simulink model "p1_digital_twin_R2023a"  (R2023a)
settings: Solver=FixedStepDiscrete  StartTime=0.0  StopTime=10  FixedStep=Ts  RelTol=1e-3  EnableMultiTasking=on
values from neighbouring files (symbols this model uses):
  ack = 1    [SteeringController.m]
  cpr_handwheel = 500*4    (= 2000)    [p1_params_new.m]
  cpr_steering = 1000*4    (= 4000)    [p1_params_new.m]
  hal_filter_den = [1 1*(2*pi*Ts)-1]    [SteeringController.m]    (also in p1_params_new.m = DEN_cellarray{1})
  hal_filter_num = [1*(2*pi*Ts)]    [SteeringController.m]    (also in p1_params_new.m = NUM_cellarray{1})
  n_drive = 5.6    [p1_params_new.m]
  n_handwheel = 50    [p1_params_new.m]
  n_steering = 160    [p1_params_new.m]
  sr = 7.5    [SteeringController.m]
  steering_limit = 35    [SteeringController.m]
  Ts = 0.001    [p1_params_new.m]
  wc = 10    [SteeringController.m]    (also in p1_params_new.m = p1params.input.VAccelFc*(2*Ts))
undefined symbols (not defined in the file or in its folder): DiscIntNeverNeededParam, p1params, param
libraries: simulink x7
(part 1 of 4)
settings Model: ExtModeTrigDuration=2  Creator=cbeal  LastModifiedBy=12406
settings SolverCC: InitialStep=.001  ZeroCrossAlgorithm=Adaptive  AlgebraicLoopSolver=TrustRegion  PositivePriorityOrder=on
settings DataIOCC: SaveFormat=Array  SignalLoggingSaveFormat=ModelDataLogs  SignalLogging=off  ReturnWorkspaceOutputs=off  Refine=5
settings OptimizationCC: EnhancedBackFolding=on  PassReuseOutputArgsAs=Individual arguments  ExpressionDepthLimit=2147483647  ZeroExternalMemoryAtStartup=off  ZeroInternalMemoryAtStartup=off  MaxStackSize=64  OptimizeBlockOrder=speed  DifferentSizesBufferReuse=on  OptimizationCustomize=off  EfficientTunableParamExpr=on
settings DebuggingCC: UnderspecifiedInitializationDetection=Classic  MergeDetectMultiDrivingBlocksExec=none  InheritedTsInSrcMsg=none  ParameterTunabilityLossMsg=error  FcnCallInpInsideContextMsg=warning  UnconnectedInputMsg=warning  UnconnectedOutputMsg=warning  UnconnectedLineMsg=warning  StateNameClashWarn=warning  SFUnexpectedBacktrackingDiag=warning  SFNoUnconditionalDefaultTransitionDiag=warning  ArithmeticOperatorsInVariantConditions=warning
settings HardwareCC: ProdBitPerPointer=32  ProdBitPerSizeT=32  ProdBitPerPtrDiffT=32  ProdLargestAtomicInteger=Long  ProdLargestAtomicFloat=Double  ProdWordSize=32  ProdLongLongMode=on  ProdHWDeviceType=ARM Compatible->ARM Cortex
settings ModelReferenceCC: EnableRefExpFcnMdlSchedulingChecks=on  PropagateSignalLabelsOutOfModel=off
settings SFSimCC: SimUseLocalCustomCode=off  CustomCodeUndefinedFunction=UseInterfaceOnly
settings RTWCC: Description=Embedded Coder  SystemTargetFile=ert.tlc  HardwareBoard=Raspberry Pi  TLCOptions="-aInlineSetEventsForThisBaseRateFcn=TLC_FALSE -aSuppressMultiTaskScheduler=TLC_FALSE  -aRateBasedStepFcn=0"  TemplateMakefile=ert_default_tmf  RTWUseLocalCustomCode=off  Toolchain=GNU GCC Embedded Linux  BuildConfiguration=Faster Runs
settings CodeAppCC: ForceParamTrailComments=on  IgnoreCustomStorageClasses=off  OperatorAnnotations=on  SimulinkDataObjDesc=on  SFDataObjDesc=on  InsertBlockDesc=on
settings ERTTargetCC: SupportVariableSizeSignals=on  ExtModeTransport=2  ExtModeStaticAlloc=on  ExtModeMexFile=ext_xcp  ExtModeIntrfLevel=Level2 - Open
settings ConfigComp: CovMetricSettings=dw  CovSaveCumulativeToWorkspaceVar=on  CovSaveSingleToWorkspaceVar=on  CovExternalEMLEnable=off

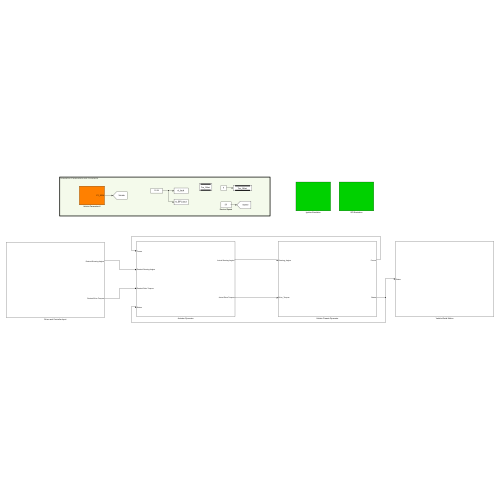
[thumbnail: Simulink's stored preview of the top-level diagram]
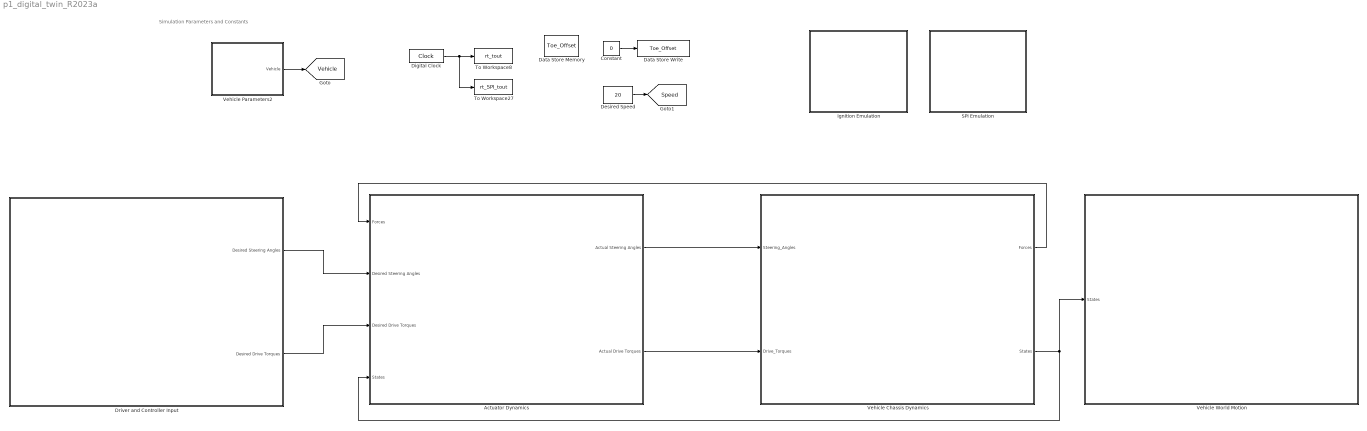
== system p1_digital_twin_R2023a ==
  note: Simulation Parameters and Constants
  Actuator Dynamics : Subsystem
  Constant : Constant  Value=0
  Data Store Memory : DataStoreMemory  DataStoreName=Toe_Offset  WriteAfterWriteMsg=warning  ShowAdditionalParam=off
  Data Store Write : DataStoreWrite  DataStoreName=Toe_Offset  IndexOptions=Index vector (dialog)  Indices=1  OutputSizes=1
  Desired Speed : Constant  Value=20
  Digital Clock : DigitalClock  SampleTime=-1
  Driver and Controller Input : Subsystem
  Ignition Emulation : Subsystem
  SPI Emulation : Subsystem
  To Workspace27 : ToWorkspace  VariableName=rt_SPI_tout  SampleTime=-1
      settings: Save2DSignal=2-D array (concatenate along first dimension)
  To Workspace8 : ToWorkspace  VariableName=rt_tout  SampleTime=-1
      settings: Save2DSignal=2-D array (concatenate along first dimension)
  Vehicle Chassis Dynamics : Subsystem
  Vehicle Parameters2 : Subsystem  mask{vehicleName='P1_2024', m=1467, m_s=1467, Ixx=0, Iyy=0, Izz=2235, Iw=1.2, Re=0.32, a=1.02, b=1.45, d=1.3, h_cg=0.42, h_rcf=0, h_rcr=0, k_phi=0, b_phi=0, Ca=[50000; 50000; 35000; 35000], Cx=[30000; 30000; 30000; 30000], mu_peak=[1.2 1.2 1.2 1.2], mu_slide=[0.9 0.9 0.9 0.9]}
      mask prompts: vehicleName "Name of Vehicle"; m "Mass"; m_s "Sprung Mass"; Ixx "Roll Moment of Inertia"; Iyy "Pitch Moment of Inertia"; Izz "Yaw Moment of Inertia"; Iw "Wheel Moment of Inertia"; Re "Wheel Effective Radius"; a "CG-Front Axle Distance"; b "CG-Rear Axle Distance"; d "Track Width"; h_cg "CG height"; h_rcf "Front Roll Center Height"; h_rcr "Rear Roll Center Height"; k_phi "Chassis Roll Stiffness (x2)"; b_phi "Chassis Roll Damping (x2)"; Ca "Cornering Stiffnesses (x4)"; Cx "Longitudinal Stiffnesses (x4)"; mu_peak "Peak Coeff. Friction (x4)"; mu_slide "Sliding Coeff. Friction (x4)"
      mask Display: port_label('output',1,vehicleName)
  Vehicle World Motion : Subsystem
  tag scope: Speed=global, Vehicle=global
  wires:
  Vehicle Parameters2/1(Vehicle) -> [Vehicle]
  Digital Clock/1 -> To Workspace27/1, To Workspace8/1
  Desired Speed/1 -> [Speed]
  Driver and Controller Input/1(Desired Steering Angles) -> Actuator Dynamics/2(Desired Steering Angles)
  Driver and Controller Input/2(Desired Drive Torques) -> Actuator Dynamics/3(Desired Drive Torques)
  Constant/1 -> Data Store Write/1
  Actuator Dynamics/1(Actual Steering Angles) -> Vehicle Chassis Dynamics/1(Steering_Angles)
  Vehicle Chassis Dynamics/2(States) -> Actuator Dynamics/4(States), Vehicle World Motion/1(States)
  Vehicle Chassis Dynamics/1(Forces) -> Actuator Dynamics/1(Forces)
  Actuator Dynamics/2(Actual Drive Torques) -> Vehicle Chassis Dynamics/2(Drive_Torques)

== system p1_digital_twin_R2023a/Actuator Dynamics ==
  Forces : Inport
  Desired Steering Angles : Inport  Port=2
  Desired Drive Torques : Inport  Port=3
  States : Inport  Port=4
  Bus Selector : BusSelector  OutputSignals=Fy
  Bus Selector1 : BusSelector  OutputSignals=Yaw Rate
  Constant : Constant  Value=0
  Drivetrain Emulation : Subsystem
  Left Steering Model : Subsystem
  Mux : Mux
  Right Steering Model : Subsystem
  Selector : Selector  InputPortWidth=4  IndexOptions=Index vector (dialog)  Indices=[1]  OutputSizes=1
  Selector1 : Selector  InputPortWidth=4  IndexOptions=Index vector (dialog)  Indices=2  OutputSizes=1
  Steering System Emulation : Subsystem
  Actual Steering Angles : Outport
  Actual Drive Torques : Outport  Port=2
  wires:
  Right Steering Model/1(delta_right) -> Mux/2  "Right"
  Left Steering Model/2(steering_left) -> Steering System Emulation/1(Left Wheel)
  Right Steering Model/2(steering_right) -> Steering System Emulation/2(Right Wheel)
  Selector/1 -> Left Steering Model/2(In2)
  Selector1/1 -> Right Steering Model/2(In2)
  Desired Steering Angles/1 -> Selector1/1, Selector/1
  Left Steering Model/1(delta_left) -> Mux/1  "Left"
  Constant/1 -> Mux/4, Mux/3
  Mux/1 -> Actual Steering Angles/1
  Bus Selector/1 -> Right Steering Model/1(Fy), Left Steering Model/1(Fy)  "<Fy>"
  Desired Drive Torques/1 -> Actual Drive Torques/1
  [Speed] -> Drivetrain Emulation/1(Vehicle Speed)
  Forces/1 -> Bus Selector/1
  States/1 -> Bus Selector1/1
  Bus Selector1/1 -> Drivetrain Emulation/2(Vehicle Yaw Rate)  "<Yaw Rate>"

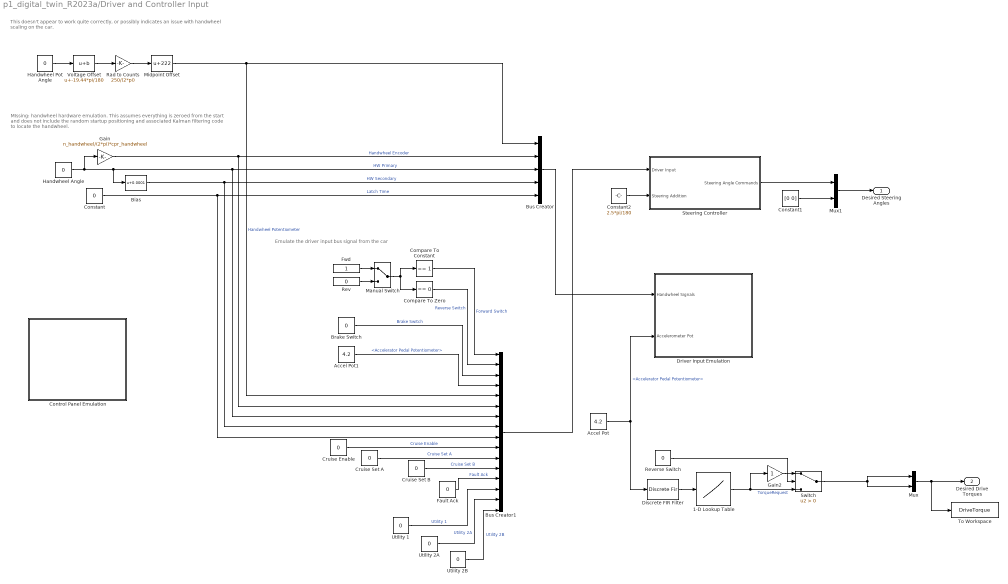
== system p1_digital_twin_R2023a/Driver and Controller Input ==
  note: Emulate the driver input bus signal from the car
  note: This doesn't appear to work quite correctly, or possibly indicates
      | an issue with handwheel scaling on the car.
  note: MIssing: handwheel hardware emulation. This assumes
      | everything is zeroed from the start and does not include the
      | random startup positioning and associated Kalman filtering
      | code to locate the handwheel.
  1-D Lookup Table : Lookup_n-D  NumberOfTableDimensions=1  BreakpointsForDimension1="[0 p1params.input.VminAccel p1params.input.VmidAccel-p1params.input.Vdeadband/2  p1params.input.VmidAccel+p1params.input.Vdeadband/2 p1params.input.VmaxAccel 5]"  Table=[p1params.input.TmaxAccel p1params.input.TmaxAccel 0 0 p1params.input.TminAccel p1params.input.TminAccel]  InternalRulePriority=Speed  RndMeth=Simplest
  Accel Pot : Constant  Value=4.2
  Accel Pot1 : Constant  Value=4.2
  Bias : Bias  Bias=0.0001  SaturateOnIntegerOverflow=off
  Brake Switch : Constant  Value=0
  Bus Creator : BusCreator  Inputs=5
  Bus Creator1 : BusCreator  Inputs=16
  Compare To Constant : simulink/Logic and Bit Operations/Compare To Constant  relop===  const=1  OutDataTypeStr=uint8
  Compare To Zero : simulink/Logic and Bit Operations/Compare To Zero  relop===  OutDataTypeStr=uint8
  Constant : Constant  Value=0
  Constant1 : Constant  Value=[0 0]
  Constant2 : Constant  Value=2.5*pi/180
  Control Panel Emulation : Subsystem
  Cruise Enable : Constant  Value=0
  Cruise Set A : Constant  Value=0
  Cruise Set B : Constant  Value=0
  Discrete FIR Filter : DiscreteFir  Coefficients=[ones(1,20)/20]
  Driver Input Emulation : Subsystem
  Fault Ack : Constant  Value=0
  Fwd : Constant
  Gain : Gain  Gain=n_handwheel/(2*pi)*cpr_handwheel
  Gain2 : Gain
  Handwheel Angle : Constant  Value=0
  Handwheel Pot Angle : Constant  Value=0
  Manual Switch : ManualSwitch
  Midpoint Offset : Bias  Bias=222  SaturateOnIntegerOverflow=off
  Mux : Mux  Inputs=2
  Mux1 : Mux  Inputs=2
  Rad to Counts : Gain  Gain=250/(2*pi)
  Rev : Constant  Value=0
  Reverse Switch : Constant  Value=0
  Steering Controller : Subsystem
      mask init:
      | p1_params_new;
      | SteeringController;
  Switch : Switch  Criteria=u2 > Threshold  SaturateOnIntegerOverflow=off  InputSameDT=off
  To Workspace : ToWorkspace  VariableName=DriveTorque  SampleTime=-1
      settings: Save2DSignal=2-D array (concatenate along first dimension)
  Utility 1 : Constant  Value=0
  Utility 2A : Constant  Value=0
  Utility 2B : Constant  Value=0
  Voltage Offset : Bias  Bias=-19.44*pi/180  SaturateOnIntegerOverflow=off
  Desired Steering Angles : Outport
  Desired Drive Torques : Outport  Port=2
  wires:
  Bus Creator/1 -> Driver Input Emulation/1(Handwheel Signals)
  Constant/1 -> Bus Creator1/9, Bus Creator/5  "Latch Time"
  Midpoint Offset/1 -> Bus Creator1/5, Bus Creator/1  "Handwheel Potentiometer"
  Handwheel Angle/1 -> Bus Creator1/7, Bus Creator/3, Bias/1, Gain/1  "HW Primary"
  Voltage Offset/1 -> Rad to Counts/1
  Handwheel Pot Angle/1 -> Voltage Offset/1
  Bias/1 -> Bus Creator1/8, Bus Creator/4  "HW Secondary"
  Rad to Counts/1 -> Midpoint Offset/1
  Gain/1 -> Bus Creator1/6, Bus Creator/2  "Handwheel Encoder"
  Mux1/1 -> Desired Steering Angles/1
  1-D Lookup Table/1 -> Switch/3, Gain2/1  "TorqueRequest"
  Reverse Switch/1 -> Switch/2
  Accel Pot/1 -> Discrete FIR Filter/1, Driver Input Emulation/2(Accelerometer Pot)  "<Accelerator Pedal Potentiometer>"
  Gain2/1 -> Switch/1
  Discrete FIR Filter/1 -> 1-D Lookup Table/1
  Mux/1 -> To Workspace/1, Desired Drive Torques/1
  Switch/1 -> Mux/2, Mux/1
  Constant1/1 -> Mux1/2
  Constant2/1 -> Steering Controller/2(Steering Addition)
  Steering Controller/1(Steering Angle Commands) -> Mux1/1
  Bus Creator1/1 -> Steering Controller/1(Driver Input)
  Fwd/1 -> Manual Switch/1
  Rev/1 -> Manual Switch/2
  Manual Switch/1 -> Compare To Zero/1, Compare To Constant/1
  Brake Switch/1 -> Bus Creator1/3  "Brake Switch"
  Accel Pot1/1 -> Bus Creator1/4  "<Accelerator Pedal Potentiometer>"
  Utility 2B/1 -> Bus Creator1/16  "Utility 2B"
  Utility 2A/1 -> Bus Creator1/15  "Utility 2A"
  Utility 1/1 -> Bus Creator1/14  "Utility 1"
  Fault Ack/1 -> Bus Creator1/13  "Fault Ack"
  Cruise Set B/1 -> Bus Creator1/12  "Cruise Set B"
  Cruise Set A/1 -> Bus Creator1/11  "Cruise Set A"
  Cruise Enable/1 -> Bus Creator1/10  "Cruise Enable"
  Compare To Zero/1 -> Bus Creator1/2  "Reverse Switch"
  Compare To Constant/1 -> Bus Creator1/1  "Forward Switch"

== system p1_digital_twin_R2023a/Ignition Emulation ==
  note: This is just a single signal that comes from the MCU. It will always
      | be on if we're taking data, so emulate it as a constant 1.
  Constant : Constant  OutDataTypeStr=uint8  SampleTime=-1
  To Workspace22 : ToWorkspace  VariableName=rt_Ignition  SampleTime=-1
      settings: Save2DSignal=2-D array (concatenate along first dimension)
  wires:
  Constant/1 -> To Workspace22/1

== system p1_digital_twin_R2023a/SPI Emulation ==
  note: Since we are not actually receiving anything over SPI in this
      | model, generate random data so that the error checking doesn't
      | flag the rest of the data as repeated (and thus erroneous).
  Constant : Constant  Value=rand(215,1)  OutDataTypeStr=double  SampleTime=-1
  Data Type Conversion : DataTypeConversion  OutDataTypeStr=uint8  SaturateOnIntegerOverflow=off  RndMeth=Floor
  Gain : Gain  Gain=255  OutDataTypeStr=double  SaturateOnIntegerOverflow=on
  Round : Rounding
  To Workspace17 : ToWorkspace  VariableName=rt_spiBytesIn  SampleTime=-1
      settings: Save2DSignal=2-D array (concatenate along first dimension)
  wires:
  Constant/1 -> Gain/1
  Round/1 -> Data Type Conversion/1
  Gain/1 -> Round/1
  Data Type Conversion/1 -> To Workspace17/1

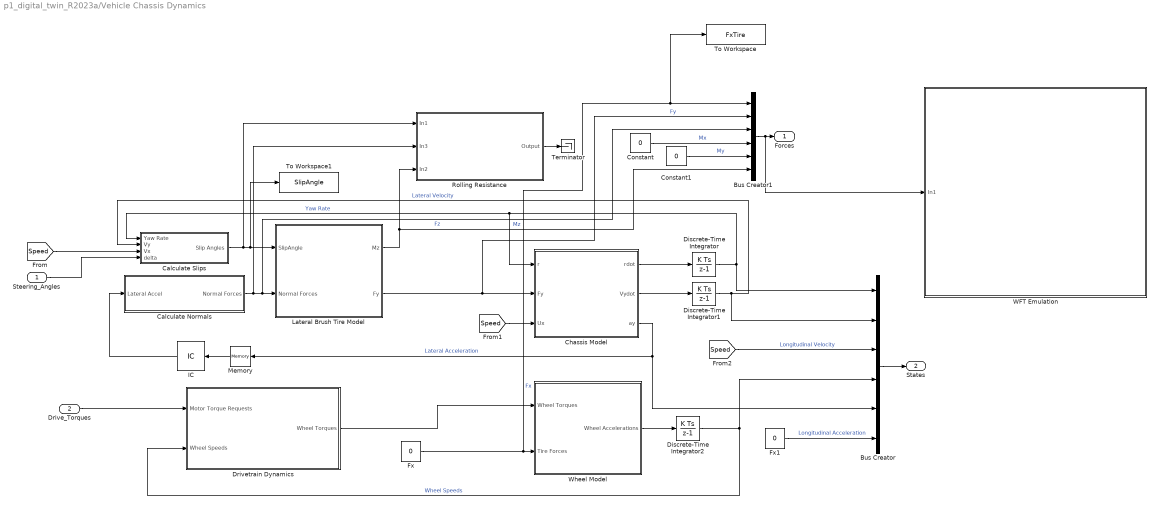
== system p1_digital_twin_R2023a/Vehicle Chassis Dynamics ==
  Steering_Angles : Inport
  Drive_Torques : Inport  Port=2
  Bus Creator : BusCreator  Inputs=6
  Bus Creator1 : BusCreator  Inputs=6
  Calculate Normals : Subsystem
  Calculate Slips : Subsystem
  Chassis Model : Subsystem
  Constant : Constant  Value=0
  Constant1 : Constant  Value=0
  Discrete-Time Integrator : DiscreteIntegrator  gainval=1  SampleTime=-1  ICPrevOutput=DiscIntNeverNeededParam  ICPrevScaledInput=DiscIntNeverNeededParam
  Discrete-Time Integrator1 : DiscreteIntegrator  gainval=1  SampleTime=-1  ICPrevOutput=DiscIntNeverNeededParam  ICPrevScaledInput=DiscIntNeverNeededParam
  Discrete-Time Integrator2 : DiscreteIntegrator  gainval=1  SampleTime=-1  ICPrevOutput=DiscIntNeverNeededParam  ICPrevScaledInput=DiscIntNeverNeededParam
  Drivetrain Dynamics : Subsystem
  Fx : Constant  Value=0
  Fx1 : Constant  Value=0
  IC : InitialCondition  Value=0
  Lateral Brush Tire Model : Subsystem
  Memory : Memory
  Rolling Resistance : Subsystem
  Terminator : Terminator
  To Workspace : ToWorkspace  VariableName=FxTire  SampleTime=-1
  To Workspace1 : ToWorkspace  VariableName=SlipAngle  SampleTime=-1
  WFT Emulation : Subsystem
  Wheel Model : Subsystem
  Forces : Outport
  States : Outport  Port=2
  wires:
  Discrete-Time Integrator/1 -> Chassis Model/1(r), Calculate Slips/1(Yaw Rate), Bus Creator/1  "Yaw Rate"
  Lateral Brush Tire Model/1(Mz) -> Bus Creator1/6, Rolling Resistance/3(In2)  "Mz"
  Chassis Model/1(rdot) -> Discrete-Time Integrator/1
  Steering_Angles/1 -> Calculate Slips/4(delta)
  IC/1 -> Calculate Normals/1(Lateral Accel)
  Calculate Normals/1(Normal Forces) -> Rolling Resistance/2(In3), Bus Creator1/3, Lateral Brush Tire Model/2(Normal Forces)  "Fz"
  Discrete-Time Integrator1/1 -> Bus Creator/2, Calculate Slips/2(Vy)  "Lateral Velocity"
  Memory/1 -> IC/1
  [Speed] -> Calculate Slips/3(Vx)
  Rolling Resistance/1(Output) -> Terminator/1
  Chassis Model/2(Vydot) -> Discrete-Time Integrator1/1
  Calculate Slips/1(Slip Angles) -> Rolling Resistance/1(In1), To Workspace1/1, Lateral Brush Tire Model/1(SlipAngle)
  Lateral Brush Tire Model/2(Fy) -> Bus Creator1/2, Chassis Model/2(Fy)  "Fy"
  Chassis Model/3(ay) -> Bus Creator/5, Memory/1  "Lateral Acceleration"
  Drive_Torques/1 -> Drivetrain Dynamics/1(Motor Torque Requests)
  Drivetrain Dynamics/1(Wheel Torques) -> Wheel Model/1(Wheel Torques)
  Wheel Model/1(Wheel Accelerations) -> Discrete-Time Integrator2/1
  Discrete-Time Integrator2/1 -> Bus Creator/4, Drivetrain Dynamics/2(Wheel Speeds)  "Wheel Speeds"
  Fx/1 -> To Workspace/1, Bus Creator1/1, Wheel Model/2(Tire Forces)  "Fx"
  [Speed] -> Chassis Model/3(Ux)
  [Speed] -> Bus Creator/3  "Longitudinal Velocity"
  Fx1/1 -> Bus Creator/6  "Longitudinal Acceleration"
  Bus Creator/1 -> States/1
  Bus Creator1/1 -> WFT Emulation/1(In1), Forces/1
  Constant/1 -> Bus Creator1/4  "Mx"
  Constant1/1 -> Bus Creator1/5  "My"

== system p1_digital_twin_R2023a/Vehicle Parameters2 ==
  Add : Sum
  Add1 : Sum
  Bus Creator : BusCreator  Inputs=21
  Constant : Constant  Value=m
  Constant1 : Constant  Value=Izz
  Constant10 : Constant  Value=Ixx
  Constant11 : Constant  Value=Iyy
  Constant12 : Constant  Value=m_s
  Constant13 : Constant  Value=Re
  Constant14 : Constant  Value=h_cg
  Constant15 : Constant  Value=h_rcf
  Constant16 : Constant  Value=h_rcr
  Constant17 : Constant  Value=k_phi
  Constant18 : Constant  Value=b_phi
  Constant2 : Constant  Value=a
  Constant3 : Constant  Value=b
  Constant4 : Constant  Value=d
  Constant5 : Constant  Value=mu_peak
  Constant6 : Constant  Value=mu_slide
  Constant7 : Constant  Value=Ca
  Constant8 : Constant  Value=Cx
  Constant9 : Constant  Value=Iw
  Gain : Gain  Gain=1/2
  Subtract : Sum  Inputs=+-
  Vehicle : Outport  VectorParamsAs1DForOutWhenUnconnected=off
  wires:
  Constant2/1 -> Add/1, Bus Creator/8  "a"
  Constant3/1 -> Add/2, Bus Creator/10  "b"
  Bus Creator/1 -> Vehicle/1
  Constant/1 -> Bus Creator/1  "m"
  Constant12/1 -> Bus Creator/2  "m_sprung"
  Constant10/1 -> Bus Creator/3  "Ixx"
  Constant11/1 -> Bus Creator/4  "Iyy"
  Constant1/1 -> Bus Creator/5  "Izz"
  Constant9/1 -> Bus Creator/6  "Iw"
  Constant13/1 -> Bus Creator/7  "Re"
  Add/1 -> Bus Creator/9  "L"
  Constant4/1 -> Bus Creator/11  "d"
  Constant14/1 -> Bus Creator/12, Subtract/1  "h_cg"
  Constant15/1 -> Bus Creator/13, Add1/1  "h_rcf"
  Constant16/1 -> Bus Creator/14, Add1/2  "h_rcr"
  Constant17/1 -> Bus Creator/16  "k_phi"
  Constant18/1 -> Bus Creator/17  "b_phi"
  Constant7/1 -> Bus Creator/18  "Ca"
  Constant8/1 -> Bus Creator/19  "Cx"
  Constant5/1 -> Bus Creator/20  "mu_peak"
  Constant6/1 -> Bus Creator/21  "mu_slide"
  Subtract/1 -> Bus Creator/15  "h1"
  Add1/1 -> Gain/1
  Gain/1 -> Subtract/2

== system p1_digital_twin_R2023a/Vehicle World Motion ==
  States : Inport
  Body Fixed to World Coords : Subsystem  mask{initialE=0, initialN=75, initialU=0, initialH=0}
      mask prompts: initialE "Initial East Coordinate"; initialN "Initial North Coordinate"; initialU "Initial Up Coordinate"; initialH "Initial Heading"
      mask Display: image('$imagefile'); % Use "Edit Image" on toolstrip to change.
  Bus Selector : BusSelector  OutputSignals=Yaw Rate,Longitudinal Acceleration,Lateral Acceleration,Lateral Velocity,Longitudinal Velocity
  Dummy : Constant  Value=0
  GPS Emulation : Subsystem
  IMU Emulation1 : Subsystem
  Road Grade : Constant  Value=0
  To Workspace : ToWorkspace  VariableName=yawrate  SampleTime=-1
  To Workspace1 : ToWorkspace  VariableName=LongVel  SampleTime=-1
  To Workspace2 : ToWorkspace  VariableName=LatVel  SampleTime=-1
  To Workspace3 : ToWorkspace  VariableName=LongAcc  SampleTime=-1
  To Workspace4 : ToWorkspace  VariableName=LatAcc  SampleTime=-1
  g : Constant  Value=-9.81
  wires:
  Body Fixed to World Coords/4(Heading) -> GPS Emulation/1(Heading)
  Body Fixed to World Coords/2(North) -> GPS Emulation/6(N)
  Bus Selector/1 -> To Workspace/1, IMU Emulation1/3(Yaw Rate), Body Fixed to World Coords/3(r)  "<Yaw Rate>"
  Body Fixed to World Coords/1(East) -> GPS Emulation/5(E)
  g/1 -> IMU Emulation1/6(Az)
  Road Grade/1 -> Body Fixed to World Coords/4(Grade)
  Bus Selector/5 -> To Workspace1/1, GPS Emulation/4(Vx), Body Fixed to World Coords/1(Vx)  "<Longitudinal Velocity>"
  Bus Selector/4 -> GPS Emulation/3(Vy), Body Fixed to World Coords/2(Vy), To Workspace2/1  "<Lateral Velocity>"
  Body Fixed to World Coords/5(Vu) -> GPS Emulation/2(Vu)
  Dummy/1 -> IMU Emulation1/2(Pitch Rate), IMU Emulation1/1(Roll Rate)
  Body Fixed to World Coords/3(Up) -> GPS Emulation/7(U)
  States/1 -> Bus Selector/1
  Bus Selector/3 -> To Workspace4/1, IMU Emulation1/5(Ay)  "<Lateral Acceleration>"
  Bus Selector/2 -> To Workspace3/1, IMU Emulation1/4(Ax)  "<Longitudinal Acceleration>"

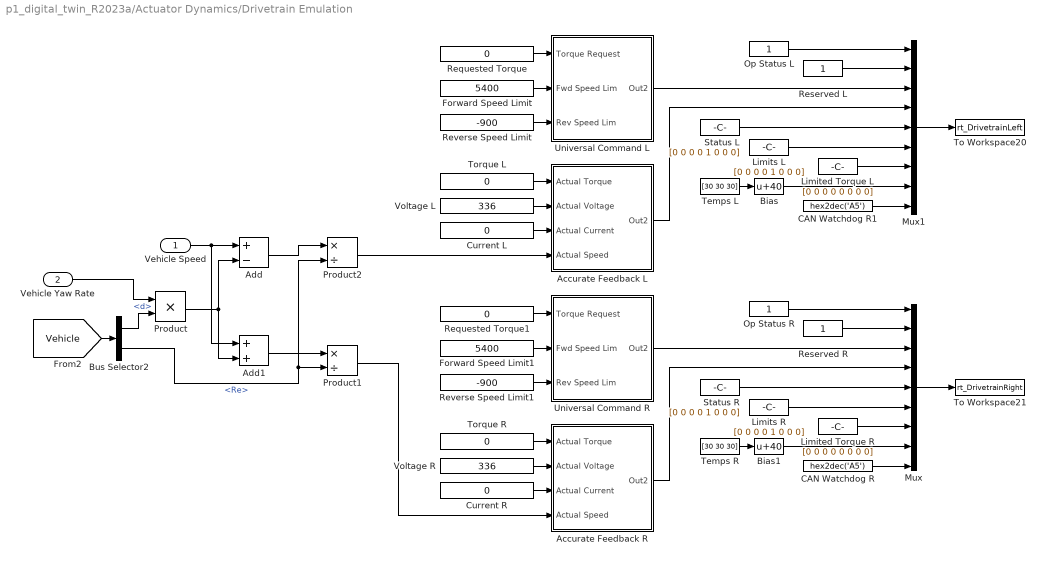
== system p1_digital_twin_R2023a/Actuator Dynamics/Drivetrain Emulation ==
  Vehicle Speed : Inport
  Vehicle Yaw Rate : Inport  Port=2
  Accurate Feedback L : Subsystem
  Accurate Feedback R : Subsystem
  Add : Sum  Inputs=+-
  Add1 : Sum
  Bias : Bias  Bias=40  SaturateOnIntegerOverflow=off
  Bias1 : Bias  Bias=40  SaturateOnIntegerOverflow=off
  Bus Selector2 : BusSelector  OutputSignals=d,Re
  CAN Watchdog R : Constant  Value=hex2dec('A5')  OutDataTypeStr=uint8  SampleTime=-1
  CAN Watchdog R1 : Constant  Value=hex2dec('A5')  OutDataTypeStr=uint8  SampleTime=-1
  Current L : Constant  Value=0  OutDataTypeStr=double  SampleTime=-1
  Current R : Constant  Value=0  OutDataTypeStr=double  SampleTime=-1
  Forward Speed Limit : Constant  Value=5400  OutDataTypeStr=double  SampleTime=-1
  Forward Speed Limit1 : Constant  Value=5400  OutDataTypeStr=double  SampleTime=-1
  Limited Torque L : Constant  Value=[0 0 0 0 0 0 0 0]  OutDataTypeStr=uint8  SampleTime=-1
  Limited Torque R : Constant  Value=[0 0 0 0 0 0 0 0]  OutDataTypeStr=uint8  SampleTime=-1
  Limits L : Constant  Value=[0 0 0 0 1 0 0 0]  OutDataTypeStr=uint8  SampleTime=-1
  Limits R : Constant  Value=[0 0 0 0 1 0 0 0]  OutDataTypeStr=uint8  SampleTime=-1
  Mux : Mux  Inputs=9
  Mux1 : Mux  Inputs=9
  Op Status L : Constant  OutDataTypeStr=uint8  SampleTime=-1
  Op Status R : Constant  OutDataTypeStr=uint8  SampleTime=-1
  Product : Product
  Product1 : Product  Inputs=*/
  Product2 : Product  Inputs=*/
  Requested Torque : Constant  Value=0  OutDataTypeStr=double  SampleTime=-1
  Requested Torque1 : Constant  Value=0  OutDataTypeStr=double  SampleTime=-1
  Reserved L : Constant  OutDataTypeStr=uint8  SampleTime=-1
  Reserved R : Constant  OutDataTypeStr=uint8  SampleTime=-1
  Reverse Speed Limit : Constant  Value=-900  OutDataTypeStr=double  SampleTime=-1
  Reverse Speed Limit1 : Constant  Value=-900  OutDataTypeStr=double  SampleTime=-1
  Status L : Constant  Value=[0 0 0 0 1 0 0 0]  OutDataTypeStr=uint8  SampleTime=-1
  Status R : Constant  Value=[0 0 0 0 1 0 0 0]  OutDataTypeStr=uint8  SampleTime=-1
  Temps L : Constant  Value=[30 30 30]  OutDataTypeStr=uint8  SampleTime=-1
  Temps R : Constant  Value=[30 30 30]  OutDataTypeStr=uint8  SampleTime=-1
  To Workspace20 : ToWorkspace  VariableName=rt_DrivetrainLeft  SampleTime=-1
  To Workspace21 : ToWorkspace  VariableName=rt_DrivetrainRight  SampleTime=-1
  Torque L : Constant  Value=0  OutDataTypeStr=double  SampleTime=-1
  Torque R : Constant  Value=0  OutDataTypeStr=double  SampleTime=-1
  Universal Command L : Subsystem
  Universal Command R : Subsystem
  Voltage L : Constant  Value=336  OutDataTypeStr=double  SampleTime=-1
  Voltage R : Constant  Value=336  OutDataTypeStr=double  SampleTime=-1
  wires:
  Mux/1 -> To Workspace21/1
  Mux1/1 -> To Workspace20/1
  Op Status R/1 -> Mux/1
  Op Status L/1 -> Mux1/1
  Reserved R/1 -> Mux/2
  Reserved L/1 -> Mux1/2
  Universal Command L/1(Out2) -> Mux1/3
  Forward Speed Limit/1 -> Universal Command L/2(Fwd Speed Lim)
  Requested Torque/1 -> Universal Command L/1(Torque Request)
  Reverse Speed Limit/1 -> Universal Command L/3(Rev Speed Lim)
  Reverse Speed Limit1/1 -> Universal Command R/3(Rev Speed Lim)
  Requested Torque1/1 -> Universal Command R/1(Torque Request)
  Forward Speed Limit1/1 -> Universal Command R/2(Fwd Speed Lim)
  Universal Command R/1(Out2) -> Mux/3
  Torque L/1 -> Accurate Feedback L/1(Actual Torque)
  Voltage L/1 -> Accurate Feedback L/2(Actual Voltage)
  Current L/1 -> Accurate Feedback L/3(Actual Current)
  [Vehicle] -> Bus Selector2/1
  Vehicle Yaw Rate/1 -> Product/1
  Bus Selector2/1 -> Product/2  "<d>"
  Torque R/1 -> Accurate Feedback R/1(Actual Torque)
  Current R/1 -> Accurate Feedback R/3(Actual Current)
  Voltage R/1 -> Accurate Feedback R/2(Actual Voltage)
  Vehicle Speed/1 -> Add1/1, Add/1
  Product/1 -> Add1/2, Add/2
  Add/1 -> Product2/1
  Add1/1 -> Product1/1
  Accurate Feedback L/1(Out2) -> Mux1/4
  Accurate Feedback R/1(Out2) -> Mux/4
  Status L/1 -> Mux1/5
  Status R/1 -> Mux/5
  Limits L/1 -> Mux1/6
  Temps L/1 -> Bias/1
  Bias/1 -> Mux1/8
  Temps R/1 -> Bias1/1
  Bias1/1 -> Mux/8
  Limits R/1 -> Mux/6
  CAN Watchdog R/1 -> Mux/9
  CAN Watchdog R1/1 -> Mux1/9
  Limited Torque R/1 -> Mux/7
  Limited Torque L/1 -> Mux1/7
  Product2/1 -> Accurate Feedback L/4(Actual Speed)
  Product1/1 -> Accurate Feedback R/4(Actual Speed)
  Bus Selector2/2 -> Product2/2, Product1/2  "<Re>"

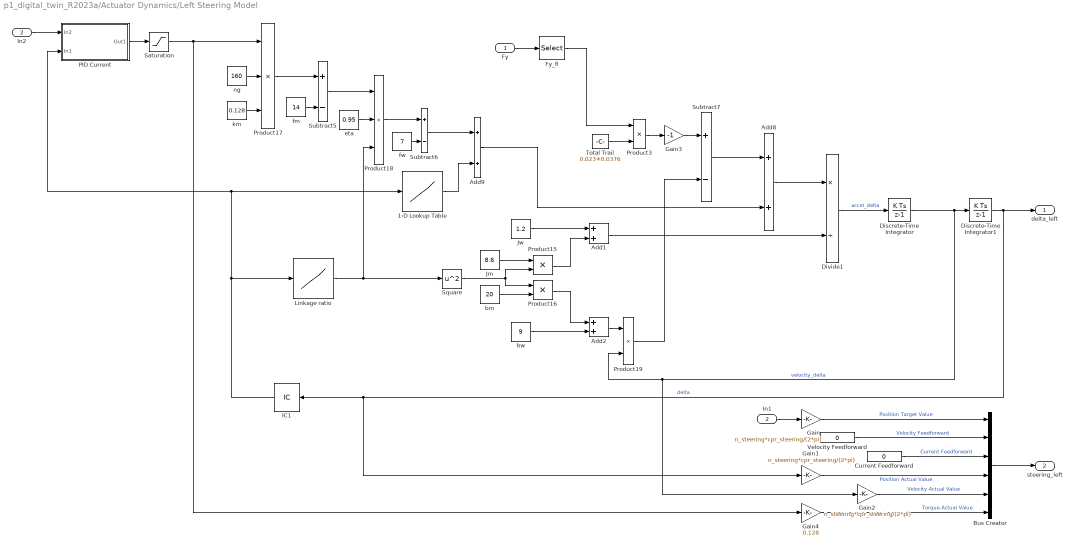
== system p1_digital_twin_R2023a/Actuator Dynamics/Left Steering Model ==
  Fy : Inport
  In2 : Inport  Port=2
  1-D Lookup Table : Lookup_n-D  NumberOfTableDimensions=1  BreakpointsForDimension1="[-0.847820835926739\t-0.827107205796427\t-0.806534902034127\t-0.786110292500230\t-0.765838938645242\t-0.745725637768374\t-0.725774464401785\t-0.705988810820495\t-0.686371426677973\t-0.666924457767370\t-0.647649483908435\t-0.628547555960088\t-0.609619231958654\t-0.590864612381775\t-0.572283374537973\t-0.553874806081885\t-0.535637837655163\t-0.517571074653039\t-0.499672828116550\t-0.481941144750437\t-0.464373836066698\t-0.446968506653820\t-0.429722581571659\t-0.412633332872000\t-0.395697905244773\t-0.378913340789940\t-0.362276602915039\t-0.345784599358402\t-0.329434204338033\t-0.313222279826152\t-0.297145695949401\t-0.281201350514722\t-0.265386187660895\t-0.249697215635740\t-0.234131523698985\t-0.218686298150805\t-0.203358837486016\t-0.188146566673940\t-0.173047050563936\t-0.158058006416590\t-0.143177315560578\t-0.128403034175186\t-0.113733403198503\t-0.0991668573612711\t-0.0847020333464052\t-0.0703377770741785\t-0.0560731501130700\t-0.0419074352162784\t-0.0278401409839011\t-0.0138710056507779\t0\t0.0137726705979163\t0.0274465650201908\t0.0410210061012758\t0.0544950812166869\t0.0678676437411695\t0.0811373153811999\t0.0943024893818217\t0.107361334607817\t0.120311800499212\t0.133151622901118\t0.145878330767912\t0.158489253741739\t0.170981530605368\t0.183352118609367\t0.195597803673620\t0.207715211463181\t0.219700819338458\t0.231550969179735\t0.243261881086027\t0.254829667948274\t0.266250350896865\t0.277519875623500\t0.288634129577384\t0.299588960035764\t0.310380193048790\t0.321003653258718\t0.331455184593447\t0.341730671834387\t0.351826063058673\t0.361737392955696\t0.371460807017988\t0.380992586606428\t0.390329174889792\t0.399467203658631\t0.408403521013489\t0.417135219927455\t0.425659667683047\t0.433974536183436\t0.442077833138002\t0.449967934122223\t0.457643615511903\t0.465104088291734\t0.472349032738191\t0.479378633976765\t0.486193618413526\t0.492795291041029\t0.499185573618547\t0.505367043726644\t0.511342974696081\t0.517117376411056]"  Table="[59.6324309072999\t57.4978468097473\t55.3167191173909\t53.0932316444003\t50.8315243188646\t48.5356726002740\t46.2096692160360\t43.8574081904947\t41.4826711148768\t39.0891155849983\t36.6802657152820\t34.2595046226666\t31.8300687620942\t29.3950439863005\t26.9573631963628\t24.5198054456362\t22.0849963580900\t19.6554097223595\t17.2333701248244\t14.8210564884303\t12.4205063885707\t10.0336210228993\t7.66217071824992\t5.30780086469900\t2.97203817406420\t0.656297167618172\t-1.63811319460166\t-3.90998282291205\t-6.15819381805507\t-8.38171386741640\t-10.5795897754865\t-12.7509411798382\t-14.8949544973830\t-17.0108771394821\t-19.0980120286550\t-21.1557124441311\t-23.1833772183472\t-25.1804463016847\t-27.1463967082544\t-29.0807388513715\t-30.9830132734844\t-32.8527877717287\t-34.6896549169416\t-36.4932299608854\t-38.2631491235684\t-39.9990682499085\t-41.7006618225439\t-43.3676223153452\t-44.9996598701173\t-46.5965022770976\t-48.1578952381318\t-49.6836028898736\t-51.1734085629835\t-52.6271157520889\t-54.0445492702632\t-55.4255565609149\t-56.7700091393347\t-58.0778041356663\t-59.3488659107952\t-60.5831477165754\t-61.7806333719443\t-62.9413389268152\t-64.0653142861919\t-65.1526447677187\t-66.2034525668524\t-67.2178981050413\t-68.1961812376902\t-69.1385423002869\t-70.0452629728457\t-70.9166669447982\t-71.7531203645787\t-72.5550320604296\t-73.3228535213536\t-74.0570786296463\t-74.7582431390482\t-75.4269238951924\t-76.0637377977342\t-76.6693405062361\t-77.2444248945768\t-77.7897192612807\t-78.3059853057423\t-78.7940158827909\t-79.2546325503824\t-79.6886829274152\t-80.0970378806866\t-80.4805885618457\t-80.8402433168140\t-81.1769244915272\t-81.4915651589718\t-81.7851057933515\t-82.0584909177590\t-82.3126657520013\t-82.5485728871192\t-82.7671490127389\t-82.9693217225836\t-83.1560064223041\t-83.3281033621739\t-83.4864948151835\t-83.6320424185280\t-83.7655846934953\t-83.8879347551672]"  InternalRulePriority=Speed  RndMeth=Simplest
  Add{1..2,8..9} (4 alike) : Sum
  Bus Creator : BusCreator  Inputs=6
  Current Feedforward : Constant  Value=0
  Discrete-Time Integrator : DiscreteIntegrator  gainval=1  SampleTime=-1  ICPrevOutput=DiscIntNeverNeededParam  ICPrevScaledInput=DiscIntNeverNeededParam
  Discrete-Time Integrator1 : DiscreteIntegrator  gainval=1  SampleTime=-1  ICPrevOutput=DiscIntNeverNeededParam  ICPrevScaledInput=DiscIntNeverNeededParam
  Divide1 : Product  Inputs=*/
  Fy_fl : Selector  InputPortWidth=4  IndexOptions=Index vector (dialog)  Indices=[1]  OutputSizes=1
  Gain : Gain  Gain=n_steering*cpr_steering/(2*pi)
  Gain1 : Gain  Gain=n_steering*cpr_steering/(2*pi)
  Gain2 : Gain  Gain=n_steering*cpr_steering/(2*pi)
  Gain3 : Gain  Gain=-1
  Gain4 : Gain  Gain=0.128
  IC1 : InitialCondition  Value=0
  In1 : InportShadow  Port=2
  Jm : Constant  Value=8.6
  Jw : Constant  Value=1.2
  Linkage ratio : Lookup_n-D  NumberOfTableDimensions=1  BreakpointsForDimension1="[-0.847820835926733\t-0.827107205796421\t-0.806534902034122\t-0.786110292500225\t-0.765838938645238\t-0.745725637768371\t-0.725774464401782\t-0.705988810820493\t-0.686371426677971\t-0.666924457767368\t-0.647649483908434\t-0.628547555960086\t-0.609619231958653\t-0.590864612381774\t-0.572283374537972\t-0.553874806081884\t-0.535637837655163\t-0.517571074653038\t-0.499672828116550\t-0.481941144750436\t-0.464373836066698\t-0.446968506653820\t-0.429722581571659\t-0.412633332872000\t-0.395697905244773\t-0.378913340789940\t-0.362276602915039\t-0.345784599358402\t-0.329434204338033\t-0.313222279826152\t-0.297145695949401\t-0.281201350514722\t-0.265386187660895\t-0.249697215635740\t-0.234131523698985\t-0.218686298150805\t-0.203358837486016\t-0.188146566673940\t-0.173047050563936\t-0.158058006416590\t-0.143177315560578\t-0.128403034175186\t-0.113733403198503\t-0.0991668573612710\t-0.0847020333464051\t-0.0703377770741785\t-0.0560731501130700\t-0.0419074352162784\t-0.0278401409839011\t-0.0138710056507779\t0\t0.0137726705979163\t0.0274465650201908\t0.0410210061012758\t0.0544950812166869\t0.0678676437411695\t0.0811373153811999\t0.0943024893818217\t0.107361334607817\t0.120311800499211\t0.133151622901118\t0.145878330767912\t0.158489253741739\t0.170981530605368\t0.183352118609367\t0.195597803673620\t0.207715211463181\t0.219700819338458\t0.231550969179735\t0.243261881086027\t0.254829667948274\t0.266250350896865\t0.277519875623500\t0.288634129577384\t0.299588960035764\t0.310380193048790\t0.321003653258718\t0.331455184593446\t0.341730671834387\t0.351826063058673\t0.361737392955696\t0.371460807017988\t0.380992586606428\t0.390329174889792\t0.399467203658631\t0.408403521013489\t0.417135219927454\t0.425659667683047\t0.433974536183436\t0.442077833138002\t0.449967934122223\t0.457643615511903\t0.465104088291734\t0.472349032738191\t0.479378633976764\t0.486193618413526\t0.492795291041029\t0.499185573618547 0.505367043726645 0.511342974696081 0.517117376411056]"  Table="[1.38455654224382\t1.37537170266767\t1.36573480138249\t1.35570099094720\t1.34532257940170\t1.33464908851767\t1.32372731204941\t1.31260137398466\t1.30131278679542\t1.28990050968874\t1.27840100685759\t1.26684830573166\t1.25527405522815\t1.24370758400264\t1.23217595869987\t1.22070404220461\t1.20931455189241\t1.19802811788048\t1.18686334127848\t1.17583685243937\t1.16496336921019\t1.15425575518290\t1.14372507794521\t1.13338066733141\t1.12323017367313\t1.11327962605023\t1.10353349054160\t1.09399472847595\t1.08466485468268\t1.07554399574266\t1.06663094823905\t1.05792323700817\t1.04941717339026\t1.04110791348034\t1.03298951637902\t1.02505500244329\t1.01729641153740\t1.00970486128364\t1.00227060531316\t0.994983091516803\t0.987831020295925\t0.980802402813211\t0.973884619243496\t0.967064477024586\t0.960328269108082\t0.953661832210192\t0.947050605062560\t0.940479686663083\t0.933933894526731\t0.927397822936366\t0.920855901193569\t0.914292451869452\t0.907691749055485\t0.901038076614312\t0.894315786430574\t0.887509356661729\t0.880603449988874\t0.873582971867560\t0.866433128778620\t0.859139486478984\t0.851688028252501\t0.844065213160760\t0.836258034293910\t0.828254077021481\t0.820041577243203\t0.811609479639830\t0.802947495923955\t0.794046163090835\t0.784896901669209\t0.775492073972122\t0.765825042347739\t0.755890227430172\t0.745683166390297\t0.735200571186576\t0.724440386815876\t0.713401849564289\t0.702085545257956\t0.690493467513883\t0.678629075990767\t0.666497354639808\t0.654104869955539\t0.641459829226640\t0.628572138786761\t0.615453462265341\t0.602117278838430\t0.588578941479510\t0.574855735210312\t0.560966935351642\t0.546933865774194\t0.532779957149379\t0.518530805200139\t0.504214228951770\t0.489860328982741\t0.475501545675519\t0.461172717467382\t0.446911139101246\t0.432756619876483\t0.418751541899740\t0.404940918335763\t0.391372451658214\t0.378096591900492]"  InternalRulePriority=Speed  RndMeth=Simplest
  PID Current : Subsystem
  Product{3,15..16,19} (4 alike) : Product
  Product17 : Product  Inputs=3
  Product18 : Product  Inputs=3
  Saturation : Saturate  UpperLimit=inf  LowerLimit=-inf
  Square : Math  Operator=square
  Subtract5 : Sum  Inputs=+-
  Subtract6 : Sum  Inputs=+-
  Subtract7 : Sum  Inputs=+-
  Total Trail : Constant  Value=0.023+0.0376
  Velocity Feedforward : Constant  Value=0
  bm : Constant  Value=20
  bw : Constant  Value=9
  eta : Constant  Value=0.95
  fm : Constant  Value=14
  fw : Constant  Value=7
  km : Constant  Value=0.128
  ng : Constant  Value=160
  delta_left : Outport
  steering_left : Outport  Port=2
  wires:
  bw/1 -> Add2/2
  fw/1 -> Subtract6/2
  Subtract7/1 -> Add8/1
  Add2/1 -> Product19/1
  Product15/1 -> Add1/2
  Saturation/1 -> Gain4/1, Product17/1
  Add9/1 -> Add8/2
  Divide1/1 -> Discrete-Time Integrator/1  "accel_delta"
  Product16/1 -> Add2/1
  In2/1 -> PID Current/1(In2)
  fm/1 -> Subtract5/2
  Add8/1 -> Divide1/1
  Subtract6/1 -> Add9/1
  Square/1 -> Product16/1, Product15/2
  Jw/1 -> Add1/1
  Discrete-Time Integrator/1 -> Discrete-Time Integrator1/1, Gain2/1, Product19/2  "velocity_delta"
  Product17/1 -> Subtract5/1
  Add1/1 -> Divide1/2
  bm/1 -> Product16/2
  Product3/1 -> Gain3/1
  ng/1 -> Product17/2
  km/1 -> Product17/3
  Linkage ratio/1 -> Square/1, Product18/3
  eta/1 -> Product18/2
  Fy/1 -> Fy_fl/1
  Product19/1 -> Subtract7/2
  Gain3/1 -> Subtract7/1
  Subtract5/1 -> Product18/1
  Product18/1 -> Subtract6/1
  Discrete-Time Integrator1/1 -> Gain1/1, IC1/1, delta_left/1  "delta"
  Jm/1 -> Product15/1
  IC1/1 -> PID Current/2(In1), 1-D Lookup Table/1, Linkage ratio/1
  Total Trail/1 -> Product3/2
  Fy_fl/1 -> Product3/1
  1-D Lookup Table/1 -> Add9/2
  In1/1 -> Gain/1
  Gain/1 -> Bus Creator/1  "Position Target Value"
  Velocity Feedforward/1 -> Bus Creator/2  "Velocity Feedforward"
  Current Feedforward/1 -> Bus Creator/3  "Current Feedforward"
  Gain1/1 -> Bus Creator/4  "Position Actual Value"
  Gain2/1 -> Bus Creator/5  "Velocity Actual Value"
  Gain4/1 -> Bus Creator/6  "Torque Actual Value"
  Bus Creator/1 -> steering_left/1
  PID Current/1(Out1) -> Saturation/1

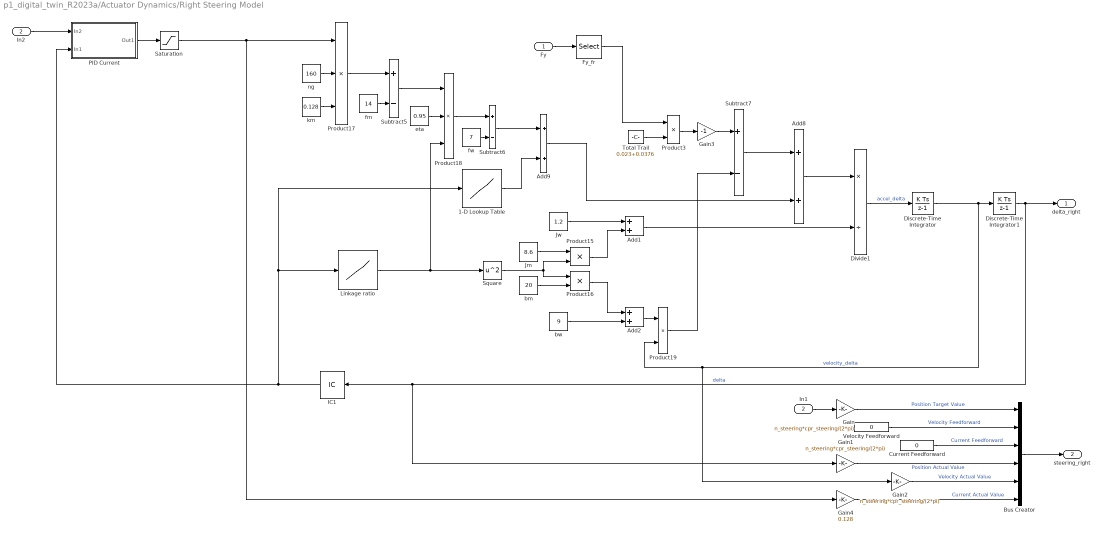
== system p1_digital_twin_R2023a/Actuator Dynamics/Right Steering Model ==
  Fy : Inport
  In2 : Inport  Port=2
  1-D Lookup Table : Lookup_n-D  NumberOfTableDimensions=1  BreakpointsForDimension1="[-0.499210914586524\t-0.494379440891288\t-0.489300972699824\t-0.483971911264309\t-0.478389639201411\t-0.472552455412233\t-0.466459511723217\t-0.460110751248000\t-0.453506848470246\t-0.446649151047424\t-0.439539623335554\t-0.432180791634912\t-0.424575691156696\t-0.416727814710647\t-0.408641063113645\t-0.400319697319244\t-0.391768292268187\t-0.382991692459873\t-0.373994969244781\t-0.364783379837862\t-0.355362328052889\t-0.345737326757763\t-0.335913962050784\t-0.325897859157887\t-0.315694650050823\t-0.305309942786319\t-0.294749292566187\t-0.284018174518396\t-0.273121958199105\t-0.262065883815657\t-0.250855040170534\t-0.239494344326268\t-0.227988522991320\t-0.216342095626912\t-0.204559359274825\t-0.192644375106154\t-0.180600956691026\t-0.168432659989277\t-0.156142775062087\t-0.143734319504583\t-0.131210033599394\t-0.118572377191172\t-0.105823528282073\t-0.0929653833481914\t-0.0799995593769682\t-0.0669273976255469\t-0.0537499691000972\t-0.0404680817560966\t-0.0270822894195731\t-0.0135929024293080\t0\t0.0136965556936115\t0.0274971037116614\t0.0414021668231140\t0.0554124322587578\t0.0695287307432392\t0.0837520138061362\t0.0980833293720719\t0.112523795629866\t0.127074573180729\t0.141736835465491\t0.156511737470876\t0.171400382714809\t0.186403788510769\t0.201522849511180\t0.216758299529836\t0.232110671643371\t0.247580256571771\t0.263167059337917\t0.278870754206175\t0.294690637900022\t0.310625581098712\t0.326673978212985\t0.342833695439807\t0.359102017096158\t0.375475590231857\t0.391950367521425\t0.408521548434989\t0.425183518688223\t0.441929787971333\t0.458752925957080\t0.475644496587836\t0.492594990641691\t0.509593756577591\t0.526628929659518\t0.543687359359710\t0.560754535040920\t0.577814509917716\t0.594849823296818\t0.611841421096472\t0.628768574644876\t0.645608797757628\t0.662337762094228\t0.678929210793610\t0.695354870388721\t0.711584361000131\t0.727585104808692\t0.743322232807229\t0.758758489831276\t0.773854137868844\t0.788566857649239]"  Table="[83.4871068797140\t83.3681200004640\t83.2380829684617\t83.0961541560951\t82.9414678860308\t82.7731365872015\t82.5902533158647\t82.3918946034474\t82.1771235884874\t81.9449933867358\t81.6945506512538\t81.4248392730637\t81.1349041724571\t80.8237951313855\t80.4905706183646\t80.1343015589392\t79.7540750069543\t79.3489976745631\t78.9181992820454\t78.4608356920374\t77.9760917966547\t77.4631841301495\t76.9213631841415\t76.3499154070360\t75.7481648739479\t75.1154746182405\t74.4512476205590\t73.7549274560427\t73.0259986050549\t72.2639864373424\t71.4684568839149\t70.6390158150929\t69.7753081470941\t68.8770167031376\t67.9438608583549\t66.9755950007592\t65.9720068431212\t64.9329156228331\t63.8581702286734\t62.7476472948450\t61.6012493037226\t60.4189027394010\t59.2005563344498\t57.9461794521723\t56.6557606462319\t55.3293064386908\t53.9668403563556\t52.5684022638386\t51.1340480299175\t49.6638495616361\t48.1578952381318\t46.6162907733789\t45.0391605339453\t43.4266493344088\t41.7789247293017\t40.0961798163247\t38.3786365610416\t36.6265496483792\t34.8402108609271\t33.0199539782800\t31.1661601854520\t29.2792639717043\t27.3597594939544\t25.4082073712637\t23.4252418687456\t21.4115784206004\t19.3680214329133\t17.2954722973813\t15.1949375373528\t13.0675369975521\t10.9145119787582\t8.73723320865886\t6.53720853031049\t4.31609018031858\t2.07568152028336\t-0.182056922464858\t-2.45500225494887\t-4.74086501391909\t-7.03718611317895\t-9.34133509909484\t-11.6505098670250\t-13.9617379843589\t-16.2718797548038\t-18.5776331430291\t-20.8755406583388\t-23.1619982703133\t-25.4332663979903\t-27.6854829768910\t-29.9146785648785\t-32.1167933983840\t-34.2876962550279\t-36.4232049172757\t-38.5191079648308\t-40.5711875514377\t-42.5752427452372\t-44.5271129314917\t-46.4227006931850\t-48.2579934995729\t-50.0290834461169\t-51.7321842023306\t-53.3636442377031]"  InternalRulePriority=Speed  RndMeth=Simplest
  Add{1..2,8..9} (4 alike) : Sum
  Bus Creator : BusCreator  Inputs=6
  Current Feedforward : Constant  Value=0
  Discrete-Time Integrator : DiscreteIntegrator  gainval=1  SampleTime=-1  ICPrevOutput=DiscIntNeverNeededParam  ICPrevScaledInput=DiscIntNeverNeededParam
  Discrete-Time Integrator1 : DiscreteIntegrator  gainval=1  SampleTime=-1  ICPrevOutput=DiscIntNeverNeededParam  ICPrevScaledInput=DiscIntNeverNeededParam
  Divide1 : Product  Inputs=*/
  Fy_fr : Selector  InputPortWidth=4  IndexOptions=Index vector (dialog)  Indices=[2]  OutputSizes=1
  Gain : Gain  Gain=n_steering*cpr_steering/(2*pi)
  Gain1 : Gain  Gain=n_steering*cpr_steering/(2*pi)
  Gain2 : Gain  Gain=n_steering*cpr_steering/(2*pi)
  Gain3 : Gain  Gain=-1
  Gain4 : Gain  Gain=0.128
  IC1 : InitialCondition  Value=0
  In1 : InportShadow  Port=2
  Jm : Constant  Value=8.6
  Jw : Constant  Value=1.2
  Linkage ratio : Lookup_n-D  NumberOfTableDimensions=1  BreakpointsForDimension1="[-0.499210914586524\t-0.494379440891288\t-0.489300972699824\t-0.483971911264309\t-0.478389639201411\t-0.472552455412234\t-0.466459511723217\t-0.460110751248000\t-0.453506848470246\t-0.446649151047424\t-0.439539623335554\t-0.432180791634913\t-0.424575691156696\t-0.416727814710648\t-0.408641063113645\t-0.400319697319244\t-0.391768292268187\t-0.382991692459873\t-0.373994969244781\t-0.364783379837862\t-0.355362328052889\t-0.345737326757763\t-0.335913962050785\t-0.325897859157887\t-0.315694650050823\t-0.305309942786319\t-0.294749292566187\t-0.284018174518396\t-0.273121958199105\t-0.262065883815657\t-0.250855040170534\t-0.239494344326268\t-0.227988522991320\t-0.216342095626912\t-0.204559359274825\t-0.192644375106154\t-0.180600956691027\t-0.168432659989277\t-0.156142775062087\t-0.143734319504583\t-0.131210033599394\t-0.118572377191172\t-0.105823528282073\t-0.0929653833481915\t-0.0799995593769683\t-0.0669273976255470\t-0.0537499691000972\t-0.0404680817560966\t-0.0270822894195731\t-0.0135929024293080\t0\t0.0136965556936115\t0.0274971037116614\t0.0414021668231140\t0.0554124322587578\t0.0695287307432392\t0.0837520138061363\t0.0980833293720719\t0.112523795629866\t0.127074573180729\t0.141736835465491\t0.156511737470876\t0.171400382714809\t0.186403788510770\t0.201522849511180\t0.216758299529836\t0.232110671643371\t0.247580256571771\t0.263167059337917\t0.278870754206175\t0.294690637900022\t0.310625581098712\t0.326673978212985\t0.342833695439807\t0.359102017096158\t0.375475590231857\t0.391950367521425\t0.408521548434989\t0.425183518688223\t0.441929787971334\t0.458752925957080\t0.475644496587836\t0.492594990641691\t0.509593756577591\t0.526628929659518\t0.543687359359710\t0.560754535040920\t0.577814509917717\t0.594849823296818\t0.611841421096473\t0.628768574644876\t0.645608797757629\t0.662337762094229\t0.678929210793611\t0.695354870388722\t0.711584361000132\t0.727585104808693\t0.743322232807231\t0.758758489831278\t0.773854137868846\t0.788566857649242]"  Table="[0.313756663598923\t0.330069397390547\t0.346656055219512\t0.363449049506934\t0.380385185830383\t0.397405548268327\t0.414455384744585\t0.431483992372781\t0.448444602800790\t0.465294267555192\t0.481993743385722\t0.498507377609720\t0.514802993456585\t0.530851775412221\t0.546628154563491\t0.562109693942666\t0.577276973871879\t0.592113477307573\t0.606605475184953\t0.620741911762434\t0.634514289966097\t0.647916556734136\t0.660944988361310\t0.673598075843394\t0.685876410221629\t0.697782567927174\t0.709320996125556\t0.720497898061121\t0.731321118401485\t0.741800028581984\t0.751945412150126\t0.761769350110043\t0.771285106266938\t0.780507012571539\t0.789450354464548\t0.798131256221094\t0.806566566295182\t0.814773742664144\t0.822770738173090\t0.830575885879361\t0.838207784396975\t0.845685183241083\t0.853026868172416\t0.860251546541738\t0.867377732634296\t0.874423633014272\t0.881407031869231\t0.888345176354574\t0.895254661937991\t0.902151317743906\t0.909050091897934\t0.915964936871325\t0.922908694825424\t0.929892982956113\t0.936928078838267\t0.944022805770202\t0.951184418118129\t0.958418486660601\t0.965728783932968\t0.973117169571823\t0.980583475659457\t0.988125392068310\t0.995738351805416\t1.00341541635686\t1.01114716103223\t1.01892156030906\t1.02672387317729\t1.03453652848370\t1.04233901027640\t1.05010774314921\t1.05781597758621\t1.06543367530608\t1.07292739460666\t1.08026017570930\t1.08739142610339\t1.09427680589076\t1.10086811313015\t1.10711316918169\t1.11295570405129\t1.11833524173512\t1.12318698556409\t1.12744170354825\t1.13102561372127\t1.13386026948490\t1.13586244495338\t1.13694402029795\t1.13701186709123\t1.13596773365175\t1.13370813038833\t1.13012421514457\t1.12510167854328\t1.11852062933098\t1.11025547972225\t1.10017483074431\t1.08814135758137\t1.07401169491911\t1.05763632228914\t1.03885944941348\t1.01751890154893\t0.993446004831594\t0.966465471621309]"  InternalRulePriority=Speed  RndMeth=Simplest
  PID Current : Subsystem
  Product{3,15..16,19} (4 alike) : Product
  Product17 : Product  Inputs=3
  Product18 : Product  Inputs=3
  Saturation : Saturate  UpperLimit=60  LowerLimit=-60
  Square : Math  Operator=square
  Subtract5 : Sum  Inputs=+-
  Subtract6 : Sum  Inputs=+-
  Subtract7 : Sum  Inputs=+-
  Total Trail : Constant  Value=0.023+0.0376
  Velocity Feedforward : Constant  Value=0
  bm : Constant  Value=20
  bw : Constant  Value=9
  eta : Constant  Value=0.95
  fm : Constant  Value=14
  fw : Constant  Value=7
  km : Constant  Value=0.128
  ng : Constant  Value=160
  delta_right : Outport
  steering_right : Outport  Port=2
  wires:
  bw/1 -> Add2/2
  fw/1 -> Subtract6/2
  Subtract7/1 -> Add8/1
  Add2/1 -> Product19/1
  Product15/1 -> Add1/2
  Add9/1 -> Add8/2
  Divide1/1 -> Discrete-Time Integrator/1  "accel_delta"
  Product16/1 -> Add2/1
  In2/1 -> PID Current/1(In2)
  fm/1 -> Subtract5/2
  Add8/1 -> Divide1/1
  Subtract6/1 -> Add9/1
  Square/1 -> Product16/1, Product15/2
  Jw/1 -> Add1/1
  Product17/1 -> Subtract5/1
  Add1/1 -> Divide1/2
  bm/1 -> Product16/2
  Product3/1 -> Gain3/1
  ng/1 -> Product17/2
  km/1 -> Product17/3
  Linkage ratio/1 -> Product18/3, Square/1
  eta/1 -> Product18/2
  Fy/1 -> Fy_fr/1
  Product19/1 -> Subtract7/2
  Gain3/1 -> Subtract7/1
  Subtract5/1 -> Product18/1
  Product18/1 -> Subtract6/1
  Jm/1 -> Product15/1
  IC1/1 -> 1-D Lookup Table/1, Linkage ratio/1, PID Current/2(In1)
  Total Trail/1 -> Product3/2
  Fy_fr/1 -> Product3/1
  1-D Lookup Table/1 -> Add9/2
  Discrete-Time Integrator/1 -> Gain2/1, Product19/2, Discrete-Time Integrator1/1  "velocity_delta"
  Gain/1 -> Bus Creator/1  "Position Target Value"
  In1/1 -> Gain/1
  PID Current/1(Out1) -> Saturation/1
  Velocity Feedforward/1 -> Bus Creator/2  "Velocity Feedforward"
  Gain4/1 -> Bus Creator/6  "Current Actual Value"
  Discrete-Time Integrator1/1 -> Gain1/1, IC1/1, delta_right/1  "delta"
  Gain1/1 -> Bus Creator/4  "Position Actual Value"
  Bus Creator/1 -> steering_right/1
  Current Feedforward/1 -> Bus Creator/3  "Current Feedforward"
  Gain2/1 -> Bus Creator/5  "Velocity Actual Value"
  Saturation/1 -> Gain4/1, Product17/1
